simulink model "trxSSB"  (R2015b)
settings: Solver=VariableStepAuto  StartTime=0.0  StopTime=10.0  RelTol=1e-3
libraries: commanapbnd3 x2, dspsrcs4 x1, dspsnks4 x1
settings Model: Creator=dominikguz  LastModifiedBy=dominikguz

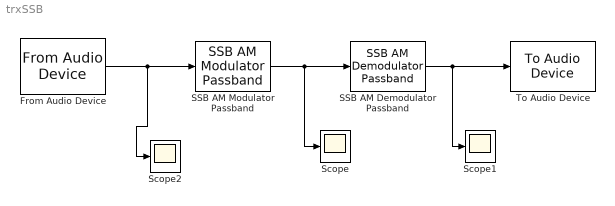
== system trxSSB ==
  From Audio Device : dspsrcs4/From Audio Device  deviceName=Default  numChannels=2  sampleRate=44100  deviceDatatype=Determine from output data type  autoBufferSize=on  bufferSize=4096  queueDuration=1.0  frameSize=1024  outputDatatype=double  defaultInputChannelMapping=on  inputChannelMapping=1:2  outputNumOverrunSamples=off  OutputFrames=off
  SSB AM Demodulator Passband : commanapbnd3/SSB AM Demodulator Passband  Fc=14000000  Ph=0  method=Butterworth  n=4  cf=14100000  Rp=0.1  Rs=50
  SSB AM Modulator Passband : commanapbnd3/SSB AM Modulator Passband  Fc=14000000  Ph=0  Sd=Upper  Ho=100
  Scope : Scope
  Scope1 : Scope
  Scope2 : Scope
  To Audio Device : dspsnks4/To Audio Device  deviceName=Default  inheritSampleRate=on  sampleRate=44100  deviceDatatype=Determine from input data type  autoBufferSize=on  bufferSize=4096  queueDuration=1.0  defaultOutputChannelMapping=on  outputChannelMapping=1:2  outputNumUnderrunSamples=off
  wires:
  SSB AM Demodulator Passband/1 -> Scope1/1, To Audio Device/1
  SSB AM Modulator Passband/1 -> Scope/1, SSB AM Demodulator Passband/1
  From Audio Device/1 -> SSB AM Modulator Passband/1, Scope2/1
